simulink model "untitled"  (Simulink 7.9)
settings: Solver=ode45  StartTime=0.0  StopTime=1000.0  RelTol=1e-3
values from neighbouring files (symbols this model uses):
  A = 10    [matlab.mat]
  B = 20    [matlab.mat]
  difK = 0    [matlab.mat]
  intK = 10    [matlab.mat]
  konK = 10    [matlab.mat]
libraries: mblibv1 x10, simulink x1
settings Model: Creator=Ivan  LastModifiedBy=Ivan
settings SimMechanicsCC: VisOnUpdateDiagram=on  VisDuringSimulation=on
settings ConfigurationSet: Description=SimMechanics 2G

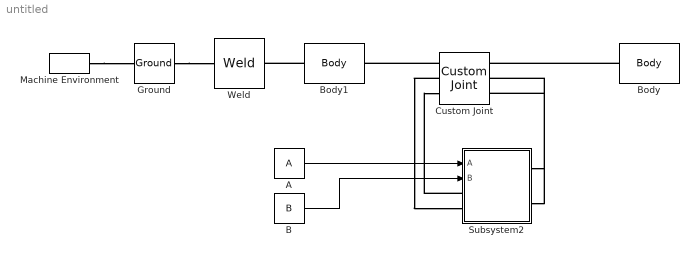
== system untitled ==
  A : Constant  Value=A
  B : Constant  Value=B
  Body : mblibv1/Bodies/Body  LConnTagsString=CS1  RConnTagsString=CS2  UpdateFromCAD=off  DialogClass=MechanicalBodyBlock  Mass=1  MassUnits=kg  InertiaUnits=kg*m^2  Inertia=eye(3)  Shape=Cylinder  ShapeDims=[1 1]  ShapeUnits=m  ShapeUse=false  Density=1  DensityUnits=kg/m^3  DensityUse=false  GraphicsMode=MACHINE_DEFAULT  BodyColorSelMode=MACHINE_DEFAULT  BodyColor=[1 0 0]  AttachedToCS=CG  CG=Left$CG$[5 0 0]$CS1$CS1$m$[0 0 0]$Euler X-Y-Z$deg$WORLD$false$none  WorkingFrames=Left$CS1$[0 0 0]$Adjoining$Adjoining$m$[0 0 0]$Euler X-Y-Z$deg$WORLD$true$none#Right$CS2$[10 0 0]$CS1$CS1$m$[0 0 0]$Euler X-Y-Z$deg$WORLD$true$none  CGPos=[5 0 0]  CGRot=[0 0 0]  CS0Pos=[]  CS0Rot=[]  CS1Pos=[0 0 0]  CS1Rot=[0 0 0]  CS2Pos=[10 0 0]  CS2Rot=[0 0 0]  CS3Pos=[]  CS3Rot=[]  CS4Pos=[]  CS4Rot=[]  CS5Pos=[]  CS5Rot=[]  CS6Pos=[]  CS6Rot=[]  CS7Pos=[]  CS7Rot=[]  CS8Pos=[]  CS8Rot=[]  CS9Pos=[]  CS9Rot=[]  CS10Pos=[]  CS10Rot=[]  CS11Pos=[]  CS11Rot=[]  CS12Pos=[]  CS12Rot=[]  CS13Pos=[]  CS13Rot=[]  CS14Pos=[]  CS14Rot=[]  CS15Pos=[]  CS15Rot=[]  CS16Pos=[]  CS16Rot=[]  CS17Pos=[]  CS17Rot=[]  CS18Pos=[]  CS18Rot=[]  CS19Pos=[]  CS19Rot=[]  CS20Pos=[]  CS20Rot=[]
  Body1 : mblibv1/Bodies/Body  LConnTagsString=CS1  RConnTagsString=CS2  UpdateFromCAD=off  DialogClass=MechanicalBodyBlock  Mass=1  MassUnits=kg  InertiaUnits=kg*m^2  Inertia=eye(3)  Shape=Cylinder  ShapeDims=[1 1]  ShapeUnits=m  ShapeUse=false  Density=1  DensityUnits=kg/m^3  DensityUse=false  GraphicsMode=MACHINE_DEFAULT  BodyColorSelMode=MACHINE_DEFAULT  BodyColor=[1 0 0]  AttachedToCS=CG  CG=Left$CG$[5 0 0]$CS1$CS1$m$[0 0 0]$Euler X-Y-Z$deg$WORLD$false$none  WorkingFrames=Left$CS1$[0 0 0]$Adjoining$Adjoining$m$[0 0 0]$Euler X-Y-Z$deg$WORLD$true$none#Right$CS2$[10 0 0]$CS1$CS1$m$[0 0 0]$Euler X-Y-Z$deg$WORLD$true$none  CGPos=[5 0 0]  CGRot=[0 0 0]  CS0Pos=[]  CS0Rot=[]  CS1Pos=[0 0 0]  CS1Rot=[0 0 0]  CS2Pos=[10 0 0]  CS2Rot=[0 0 0]  CS3Pos=[]  CS3Rot=[]  CS4Pos=[]  CS4Rot=[]  CS5Pos=[]  CS5Rot=[]  CS6Pos=[]  CS6Rot=[]  CS7Pos=[]  CS7Rot=[]  CS8Pos=[]  CS8Rot=[]  CS9Pos=[]  CS9Rot=[]  CS10Pos=[]  CS10Rot=[]  CS11Pos=[]  CS11Rot=[]  CS12Pos=[]  CS12Rot=[]  CS13Pos=[]  CS13Rot=[]  CS14Pos=[]  CS14Rot=[]  CS15Pos=[]  CS15Rot=[]  CS16Pos=[]  CS16Rot=[]  CS17Pos=[]  CS17Rot=[]  CS18Pos=[]  CS18Rot=[]  CS19Pos=[]  CS19Rot=[]  CS20Pos=[]  CS20Rot=[]
  Custom Joint : mblibv1/Joints/Custom Joint  LConnTagsString=__newl0|SA1|SA2  RConnTagsString=__newr0|SA1|SA2  UpdateFromCAD=off  NumSAPorts=4  CutJoint=off  MarkAsCut=off  Primitives=prismatic  PrimitiveProps=R1$Base$[0 0 1]$Revolute#R2$Base$[0 1 0]$Revolute  DialogClass=JointBlock  R1Axis=[0 0 1]  R2Axis=[0 1 0]  R3Axis=[]  P1Axis=[]  P2Axis=[]  P3Axis=[]  SAxis=[]
  Ground : mblibv1/Bodies/Ground  UpdateFromCAD=off  LeftPortType=env  RightPortType=workingframe  PhysicalDomain=Mechanical  DialogClass=GroundBlock  CoordPosition=[0 0 0]  CoordPositionUnits=m  StateVectorMgrId=0  MachineId=[1 0]  ShowEnvPort=on
  Machine Environment : mblibv1/Bodies/Machine Environment  PortType=env  PhysicalDomain=Mechanical  DialogTemplateClass=MECH.MachineEnvironment  SyncWhenCopied=off  Gravity=[0 -9.81 0]  GravityUnits=m/s^2  GravityAsSignal=off  Dimensionality=Auto-detect  AnalysisType=Forward dynamics  LinearAssemblyTolerance=1e-3  LinearAssemblyToleranceUnits=m  AngularAssemblyTolerance=1e-3  AngularAssemblyToleranceUnits=rad  ConstraintSolverType=Stabilizing  ConstraintRelTolerance=1e-4  ConstraintAbsTolerance=1e-4  UseRobustSingularityHandling=off  RedundancyAnalysisToleranceType=Automatically select tolerance  RedundancyAnalysisTolerance=1e-14  StatePerturbationType=Fixed  PerturbationSize=1e-5  VisualizeMachine=on  BodyVisualizationType=Use model default body geometries  BodyColorSelMode=Use model default  DefaultBodyColor=[1 0 0]
  Subsystem2 : Subsystem
  Weld : mblibv1/Joints/Weld  LConnTagsString=__newl0  RConnTagsString=__newr0  UpdateFromCAD=off  NumSAPorts=0  CutJoint=off  MarkAsCut=off  Primitives=weld  PrimitiveProps=W$WORLD$[0 0 0]$weld  DialogClass=JointBlock  WAxis=[0 0 0]
  wires:
  B/1 -> Subsystem2/2(B)
  A/1 -> Subsystem2/1(A)
  connections:
  Custom Joint/LConn2 -- Subsystem2/LConn2
  Subsystem2/LConn1 -- Custom Joint/LConn3
  Subsystem2/RConn1 -- Custom Joint/RConn3
  Subsystem2/RConn2 -- Custom Joint/RConn2
  Body/LConn1 -- Custom Joint/RConn1
  Machine Environment/RConn1 -- Ground/LConn1
  Ground/RConn1 -- Weld/LConn1
  Body1/LConn1 -- Weld/RConn1
  Custom Joint/LConn1 -- Body1/RConn1

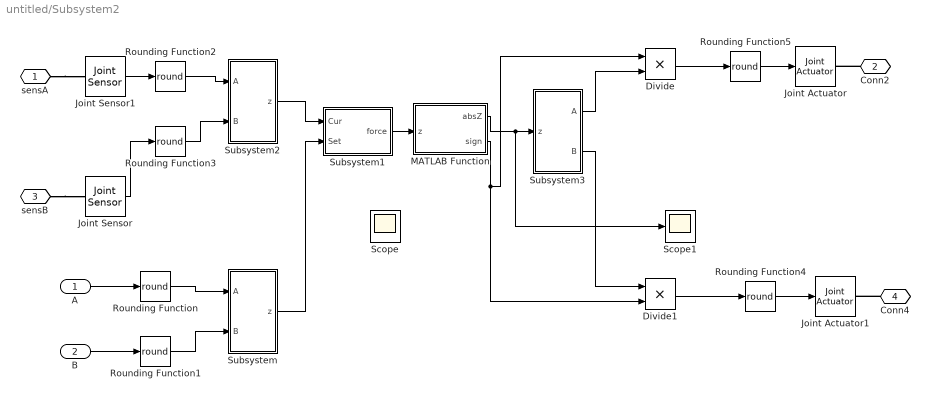
== system untitled/Subsystem2 ==
  A : Inport
  B : Inport  Port=2
  Divide : Product  Inputs=**
  Divide1 : Product  Inputs=**
  Joint Actuator : mblibv1/Sensors &  Actuators/Joint Actuator  UpdateFromCAD=off  PhysicalDomain=Mechanical  PortType=blob  ActuationStyle=Force  AngleUnits=deg  ArcVelocityUnits=deg/s  ArcAccelerationUnits=deg/s^2  CoordPositionUnits=m  VelocityUnits=m/s  AccelerationUnits=m/s^2  ForceUnits=N  TorqueUnits=N*m  ActiveIO=on  Width=1  DialogClass=MechanicalActuatorBlock  Primitive=R1  ReferenceFrame=Absolute (World)
  Joint Actuator1 : mblibv1/Sensors &  Actuators/Joint Actuator  UpdateFromCAD=off  PhysicalDomain=Mechanical  PortType=blob  ActuationStyle=Force  AngleUnits=deg  ArcVelocityUnits=deg/s  ArcAccelerationUnits=deg/s^2  CoordPositionUnits=m  VelocityUnits=m/s  AccelerationUnits=m/s^2  ForceUnits=N  TorqueUnits=N*m  ActiveIO=on  Width=1  DialogClass=MechanicalActuatorBlock  Primitive=R2  ReferenceFrame=Absolute (World)
  Joint Sensor : mblibv1/Sensors &  Actuators/Joint Sensor  UpdateFromCAD=off  PhysicalDomain=Mechanical  PortType=blob  Muxed=on  Pose=off  Angle=on  AngleUnits=deg  ArcVelocity=off  ArcVelocityUnits=deg/s  ArcAcceleration=off  ArcAccelerationUnits=deg/s^2  CoordPosition=on  CoordPositionUnits=m  Velocity=off  VelocityUnits=m/s  Acceleration=off  AccelerationUnits=m/s^2  Quaternion=on  QuaternionDT=off  QuaternionDDT=off  QuaternionUnits=off  OutputVector=[1]  ActiveIO=on  Width=1  DialogClass=MechanicalSensorBlock  Primitive=R2  Force=off  ForceUnits=N  Torque=off  TorqueUnits=N*m  ReferenceFrame=Absolute (World)  ReactionSensedSide=Base  ReactionReferenceFrame=Absolute (World)  ReactionForce=off  ReactionForceUnits=N  ReactionMoment=off  ReactionMomentUnits=N*m
  Joint Sensor1 : mblibv1/Sensors &  Actuators/Joint Sensor  UpdateFromCAD=off  PhysicalDomain=Mechanical  PortType=blob  Muxed=on  Pose=off  Angle=on  AngleUnits=deg  ArcVelocity=off  ArcVelocityUnits=deg/s  ArcAcceleration=off  ArcAccelerationUnits=deg/s^2  CoordPosition=on  CoordPositionUnits=m  Velocity=off  VelocityUnits=m/s  Acceleration=off  AccelerationUnits=m/s^2  Quaternion=on  QuaternionDT=off  QuaternionDDT=off  QuaternionUnits=off  OutputVector=[1]  ActiveIO=on  Width=1  DialogClass=MechanicalSensorBlock  Primitive=R1  Force=off  ForceUnits=N  Torque=off  TorqueUnits=N*m  ReferenceFrame=Absolute (World)  ReactionSensedSide=Base  ReactionReferenceFrame=Absolute (World)  ReactionForce=off  ReactionForceUnits=N  ReactionMoment=off  ReactionMomentUnits=N*m
  MATLAB Function : MATLAB Function  TreatAsAtomicUnit=on
  Rounding Function{,1..5} (6 alike) : Rounding  Operator=round
  Scope : Scope
      settings: YMin=-7500  YMax=15000
  Scope1 : Scope
      settings: YMin=0  YMax=100000  SaveName=ScopeData2
  Subsystem : Subsystem
  Subsystem1 : Subsystem
  Subsystem2 : Subsystem
  Subsystem3 : Subsystem
  sensA : PMIOPort  Port=1  Side=Left
  Conn2 : PMIOPort  Port=2  Side=Right
  sensB : PMIOPort  Port=3  Side=Left
  Conn4 : PMIOPort  Port=4  Side=Right
  wires:
  Subsystem2/1(z) -> Subsystem1/1(Cur)
  Subsystem/1(z) -> Subsystem1/2(Set)
  Joint Sensor/1 -> Rounding Function3/1
  Joint Sensor1/1 -> Rounding Function2/1
  Rounding Function2/1 -> Subsystem2/1(A)
  Rounding Function3/1 -> Subsystem2/2(B)
  A/1 -> Rounding Function/1
  B/1 -> Rounding Function1/1
  Rounding Function/1 -> Subsystem/1(A)
  Rounding Function1/1 -> Subsystem/2(B)
  Rounding Function4/1 -> Joint Actuator1/1
  Rounding Function5/1 -> Joint Actuator/1
  Subsystem1/1(force) -> MATLAB Function/1(z)
  MATLAB Function/1(absZ) -> Subsystem3/1(z), Scope1/1
  MATLAB Function/2(sign) -> Divide1/2, Divide/1
  Subsystem3/1(A) -> Divide/2
  Subsystem3/2(B) -> Divide1/1
  Divide/1 -> Rounding Function5/1
  Divide1/1 -> Rounding Function4/1
  connections:
  sensA/RConn1 -- Joint Sensor1/LConn1
  Conn2/RConn1 -- Joint Actuator/RConn1
  sensB/RConn1 -- Joint Sensor/LConn1
  Conn4/RConn1 -- Joint Actuator1/RConn1

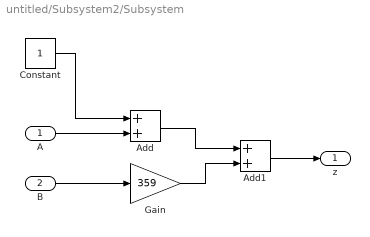
== system untitled/Subsystem2/Subsystem ==
  A : Inport
  B : Inport  Port=2
  Add : Sum
  Add1 : Sum
  Constant : Constant
  Gain : Gain  Gain=359
  z : Outport
  wires:
  B/1 -> Gain/1
  A/1 -> Add/2
  Constant/1 -> Add/1
  Add/1 -> Add1/1
  Gain/1 -> Add1/2
  Add1/1 -> z/1

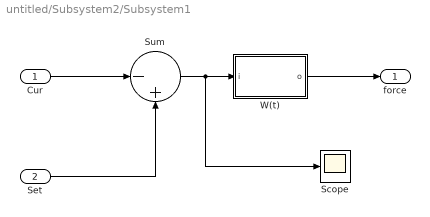
== system untitled/Subsystem2/Subsystem1 ==
  Cur : Inport
  Set : Inport  Port=2
  Scope : Scope
      settings: YMin=-7500  YMax=15000
  Sum : Sum  Inputs=|-+
  W(t) : Subsystem
  force : Outport
  wires:
  Sum/1 -> W(t)/1(i), Scope/1
  Cur/1 -> Sum/1
  Set/1 -> Sum/2
  W(t)/1(o) -> force/1

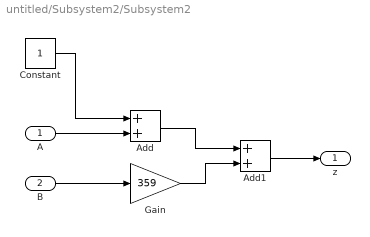
== system untitled/Subsystem2/Subsystem2 ==
  A : Inport
  B : Inport  Port=2
  Add : Sum
  Add1 : Sum
  Constant : Constant
  Gain : Gain  Gain=359
  z : Outport
  wires:
  B/1 -> Gain/1
  A/1 -> Add/2
  Constant/1 -> Add/1
  Add/1 -> Add1/1
  Gain/1 -> Add1/2
  Add1/1 -> z/1

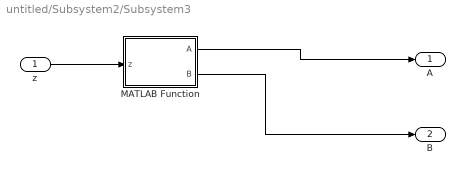
== system untitled/Subsystem2/Subsystem3 ==
  z : Inport
  MATLAB Function : MATLAB Function  TreatAsAtomicUnit=on
  A : Outport
  B : Outport  Port=2
  wires:
  z/1 -> MATLAB Function/1(z)
  MATLAB Function/1(A) -> A/1
  MATLAB Function/2(B) -> B/1

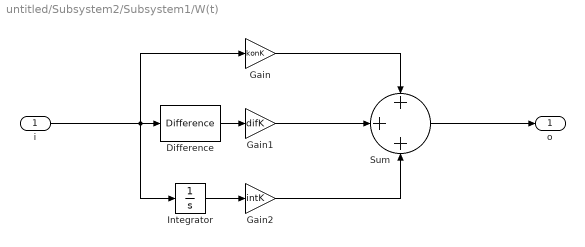
== system untitled/Subsystem2/Subsystem1/W(t) ==
  i : Inport
  Difference : simulink/Discrete/Difference  ICPrevInput=0.0  InputProcessing=Inherited  OutMin=[]  OutMax=[]  OutDataType=fixdt(1, 16)  OutScaling=2^-10  DoSatur=off
  Gain : Gain  Gain=konK
  Gain1 : Gain  Gain=difK
  Gain2 : Gain  Gain=intK
  Integrator : Integrator
  Sum : Sum  Inputs=+++
  o : Outport
  wires:
  Gain/1 -> Sum/1
  Gain1/1 -> Sum/2
  Gain2/1 -> Sum/3
  Integrator/1 -> Gain2/1
  Difference/1 -> Gain1/1
  Sum/1 -> o/1
  i/1 -> Gain/1, Difference/1, Integrator/1

== matlab function Subsystem2/MATLAB Function ==
  data: z input double; absZ output double; sign output double
function [absZ,sign] = fcn(z)
%#codegen
absZ=1;
sign=1;
if z==0
    sign=1;
    absZ=1;
end;
if z>0
    sign=1;
    absZ=abs(z);
end;
if z>0
    sign=-1;
    absZ=abs(z);
end;

== matlab function Subsystem2/Subsystem3/MATLAB Function ==
  data: z input double; A output double; B output double
function [A,B] = stats(z)
A=mod(z,359)-1;
B=(z-A-1)/359;
